simulink model "pre_lab"  (R2023b)
settings: Solver=ode4  StartTime=0.0  StopTime=5  FixedStep=1e-04  RelTol=1e-3
values from neighbouring files (symbols this model uses):
  CFP085 = (1/(2*pi*f))*(abs(Qc2)/(3*(Vc^2)))    [script.m]
  CFP095 = (1/(2*pi*f))*(abs(Qc3)/(3*(Vc^2)))    [script.m]
  CFP1 = (1/(2*pi*f))*(abs(Qc)/(3*(Vc^2)))    [script.m]
  f = 60    [script.m]
  L = XL/(omega)    (= 0.358098621957)    [script.m]
  r = 135    [script.m]
  Rc = 0.1    [script.m]
  Vl = 220    [script.m]
libraries: spsSeriesRLCBranchLib x18, spsThreePhaseBreakerLib x6, spsCurrentMeasurementLib x3, spsParallelRLCBranchLib x3, spsRMSLib x3, spsGroundLib x2, eePowerMeasurement x1, spsThreePhaseVIMeasurementLib x1, spsThreePhaseSourceLib x1, spsVoltageMeasurementLib x1, spspowerguiLib x1
settings Model: Creator=caugu  LastModifiedBy=caugu
settings ModelReferenceCC: EnableRefExpFcnMdlSchedulingChecks=on

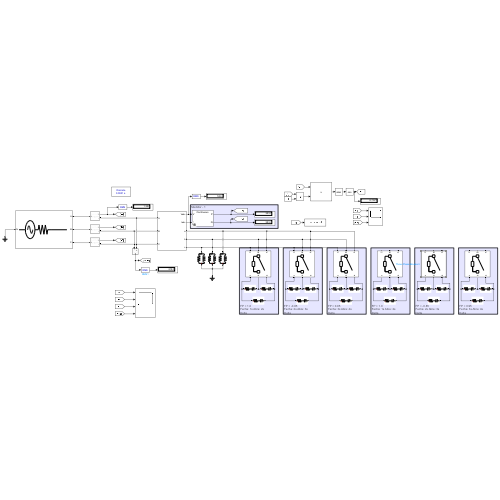
[thumbnail: Simulink's stored preview of the top-level diagram]
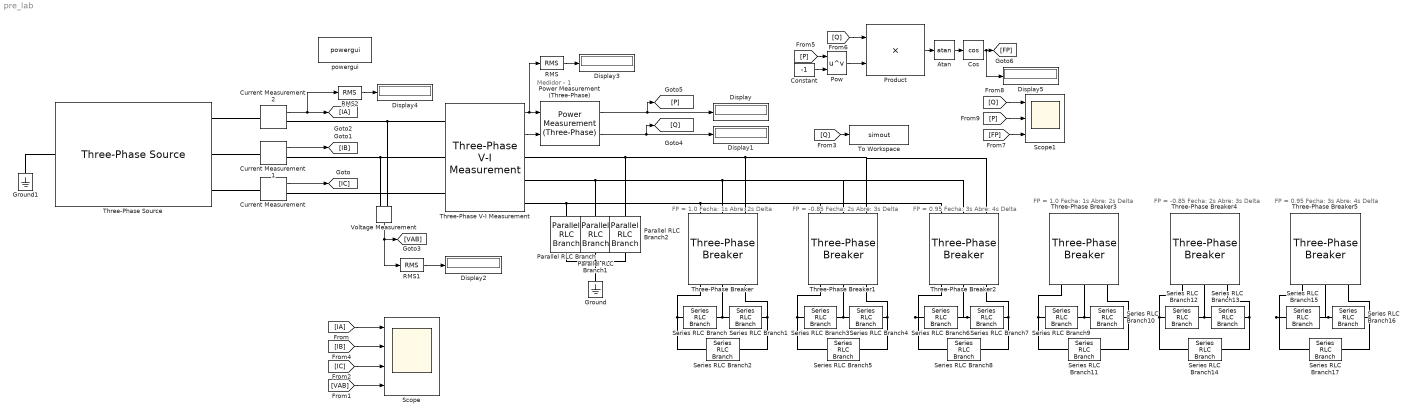
== system pre_lab ==
  note: FP = 1.0
      | Fecha: 1s Abre: 2s
      | Delta
  note: Medidor - 1
  note: FP = -0.85
      | Fecha: 2s Abre: 3s
      | Delta
  note: FP = 0.95
      | Fecha: 3s Abre: 4s
      | Delta
  note: FP = 1.0
      | Fecha: 1s Abre: 2s
      | Delta
  note: FP = -0.85
      | Fecha: 2s Abre: 3s
      | Delta
  note: FP = 0.95
      | Fecha: 3s Abre: 4s
      | Delta
  Atan : Trigonometry  Operator=atan
  Constant : Constant  Value=-1
  Cos : Trigonometry  Operator=cos
  Current Measurement : spsCurrentMeasurementLib/Current Measurement  PhasorSimulation=off  OutputType=Complex  PSBequivalent=0
  Current Measurement1 : spsCurrentMeasurementLib/Current Measurement  PhasorSimulation=off  OutputType=Complex  PSBequivalent=0
  Current Measurement2 : spsCurrentMeasurementLib/Current Measurement  PhasorSimulation=off  OutputType=Complex  PSBequivalent=0
  Display{,1..5} (6 alike) : Display
  Ground : spsGroundLib/Ground  LConnTagsString=a
  Ground1 : spsGroundLib/Ground  LConnTagsString=a
  Parallel RLC Branch : spsParallelRLCBranchLib/Parallel RLC Branch  LConnTagsString=a  RConnTagsString=__new0  BranchType=RL  Resistance=r  Inductance=L  SetiL0=off  InitialCurrent=0  Capacitance=1e-6  Setx0=off  InitialVoltage=0  Measurements=None
  Parallel RLC Branch1 : spsParallelRLCBranchLib/Parallel RLC Branch  LConnTagsString=a  RConnTagsString=__new0  BranchType=RL  Resistance=r  Inductance=L  SetiL0=off  InitialCurrent=0  Capacitance=1e-6  Setx0=off  InitialVoltage=0  Measurements=None
  Parallel RLC Branch2 : spsParallelRLCBranchLib/Parallel RLC Branch  LConnTagsString=a  RConnTagsString=__new0  BranchType=RL  Resistance=r  Inductance=L  SetiL0=off  InitialCurrent=0  Capacitance=1e-6  Setx0=off  InitialVoltage=0  Measurements=None
  Pow : Math  Operator=pow  SignedPower=on  RndMeth=Zero
  Power Measurement (Three-Phase) : eePowerMeasurement/Power Measurement (Three-Phase)  LabelModeActiveChoice=Continuous  F=60  K=[1]  Seq=Positive  Ts=0
  Product : Product
  RMS : spsRMSLib/RMS  TrueRMS=on  Freq=60  RMSInit=120  Ts=0
  RMS1 : spsRMSLib/RMS  TrueRMS=on  Freq=60  RMSInit=120  Ts=0
  RMS2 : spsRMSLib/RMS  TrueRMS=on  Freq=60  RMSInit=120  Ts=0
  Scope : Scope  NumInputPorts=4
  Scope1 : Scope  NumInputPorts=3
  Series RLC Branch{,1..2,9..11} (6 alike) : spsSeriesRLCBranchLib/Series RLC Branch  LConnTagsString=__new0  RConnTagsString=__new0  BranchType=RC  Resistance=Rc  Inductance=1e-3  SetiL0=off  InitialCurrent=0  Capacitance=CFP1  Setx0=off  InitialVoltage=0  Measurements=None
  Series RLC Branch{3..5,12..14} (6 alike) : spsSeriesRLCBranchLib/Series RLC Branch  LConnTagsString=__new0  RConnTagsString=__new0  BranchType=RC  Resistance=Rc  Inductance=1e-3  SetiL0=off  InitialCurrent=0  Capacitance=CFP085  Setx0=off  InitialVoltage=0  Measurements=None
  Series RLC Branch{6..8,15..17} (6 alike) : spsSeriesRLCBranchLib/Series RLC Branch  LConnTagsString=__new0  RConnTagsString=__new0  BranchType=RC  Resistance=Rc  Inductance=1e-3  SetiL0=off  InitialCurrent=0  Capacitance=CFP095  Setx0=off  InitialVoltage=0  Measurements=None
  Three-Phase V-I Measurement : spsThreePhaseVIMeasurementLib/Three-Phase V-I Measurement  VoltageMeasurement=phase-to-ground  SetLabelV=off  LabelV=Vabc  Vpu=off  VpuLL=off  CurrentMeasurement=yes  SetLabelI=off  LabelI=Iabc  Ipu=off  Pbase=100e6  Vbase=500e3  OutputType=Complex  PhasorSimulation=off  PSBequivalent=0
  Three-Phase Breaker : spsThreePhaseBreakerLib/Three-Phase Breaker  InitialState=open  SwitchA=on  SwitchB=on  SwitchC=on  SwitchTimes=[1 2]  External=off  BreakerResistance=0.01  SnubberResistance=1e6  SnubberCapacitance=inf  Measurements=None
  Three-Phase Breaker1 : spsThreePhaseBreakerLib/Three-Phase Breaker  InitialState=open  SwitchA=on  SwitchB=on  SwitchC=on  SwitchTimes=[2 3]  External=off  BreakerResistance=0.01  SnubberResistance=1e6  SnubberCapacitance=inf  Measurements=None
  Three-Phase Breaker2 : spsThreePhaseBreakerLib/Three-Phase Breaker  InitialState=open  SwitchA=on  SwitchB=on  SwitchC=on  SwitchTimes=[3 4]  External=off  BreakerResistance=0.01  SnubberResistance=1e6  SnubberCapacitance=inf  Measurements=None
  Three-Phase Breaker3 : spsThreePhaseBreakerLib/Three-Phase Breaker  InitialState=open  SwitchA=on  SwitchB=on  SwitchC=on  SwitchTimes=[1 2]  External=off  BreakerResistance=0.01  SnubberResistance=1e6  SnubberCapacitance=inf  Measurements=None
  Three-Phase Breaker4 : spsThreePhaseBreakerLib/Three-Phase Breaker  InitialState=open  SwitchA=on  SwitchB=on  SwitchC=on  SwitchTimes=[2 3]  External=off  BreakerResistance=0.01  SnubberResistance=1e6  SnubberCapacitance=inf  Measurements=None
  Three-Phase Breaker5 : spsThreePhaseBreakerLib/Three-Phase Breaker  InitialState=open  SwitchA=on  SwitchB=on  SwitchC=on  SwitchTimes=[3 4]  External=off  BreakerResistance=0.01  SnubberResistance=1e6  SnubberCapacitance=inf  Measurements=None
  Three-Phase Source : spsThreePhaseSourceLib/Three-Phase Source  InternalConnection=Yn  VoltagePhases=off  Voltage=Vl  PhaseAngle=0  Voltage_phases=[25e3 25e3 25e3]/sqrt(3)  PhaseAngles_phases=[0 -120 +120]  Frequency=f  NonIdealSource=on  SpecifyImpedance=off  Resistance=0.8929  Inductance=0  ShortCircuitLevel=100e6  BaseVoltage=25e3  XRratio=7  BusType=swing  Pref=10e3  Qref=0  Prefabc=[10e3, 10e3, 10e3]  Qrefabc=[0, 0, 0]  Qmin=-inf  Qmax=inf
  To Workspace : ToWorkspace  VariableName=simout  SaveFormat=Structure With Time  SampleTime=-1
  Voltage Measurement : spsVoltageMeasurementLib/Voltage Measurement  PhasorSimulation=off  OutputType=Complex  PSBequivalent=0
  powergui : spspowerguiLib/powergui  Priority=1  SimulationMode=Discrete  SampleTime=1e-4  frequency=60  Iterations=50  frequencyindice=0  Pbase=100e6  ErrMax=1e-4  UnitsV=kV  UnitsW=MW  buscounter=0  FunctionMessages=off  echomessages=off  EnableUseOfTLC=off  CurrentSourceSwitches=off  DisableSnubberDevices=off  DisableRonSwitches=off  DisableVfSwitches=off  DisplayEquations=off  AutomaticDiscreteSolvers=off  SolverType=Tustin/Backward Euler (TBE)  Interpol=off  ExternalGateDelay=off  methode=off  Ts=100  x0status=blocks  SPID=on  SwTol=0  HookPort=off  NonlinearTolerance=1e-4  nMaxIteration=100  ContinueOnMaxIteration=off  RestoreLinks=warning  ResistiveCurrentMeasurement=off  Frange=[0:2:500]  Ylog=off  Xlog=on  ShowGrid=off  save=off  variable=ZData  structure=0  ZoomFFT=off  StartTime=0.0  cycles=1  DisplayStyle=1  fundamental=60  FreqAxis=off  MaxFrequency=1000  frequencyindicesteady=1  RmsSteady=1  display=off
  wires:
  Current Measurement2/1 -> RMS2/1, [IA]
  Current Measurement1/1 -> [IB]
  Current Measurement/1 -> [IC]
  Voltage Measurement/1 -> RMS1/1, [VAB]
  Three-Phase V-I Measurement/1 -> RMS/1, Power Measurement (Three-Phase)/1
  Three-Phase V-I Measurement/2 -> Power Measurement (Three-Phase)/2
  Power Measurement (Three-Phase)/1 -> [P], Display/1
  Power Measurement (Three-Phase)/2 -> [Q], Display1/1
  [IA] -> Scope/1
  [VAB] -> Scope/4
  [IC] -> Scope/3
  [Q] -> To Workspace/1
  [IB] -> Scope/2
  RMS/1 -> Display3/1
  RMS1/1 -> Display2/1
  RMS2/1 -> Display4/1
  [FP] -> Scope1/3
  [Q] -> Scope1/1
  [P] -> Scope1/2
  Constant/1 -> Pow/2
  [P] -> Pow/1
  [Q] -> Product/1
  Pow/1 -> Product/2
  Product/1 -> Atan/1
  Atan/1 -> Cos/1
  Cos/1 -> Display5/1, [FP]
  connections:
  Current Measurement2/LConn1 -- Three-Phase Source/RConn1
  Three-Phase Source/RConn2 -- Current Measurement1/LConn1
  Three-Phase Source/RConn3 -- Current Measurement/LConn1
  Current Measurement2/RConn1 -- Voltage Measurement/LConn1 -- Three-Phase V-I Measurement/LConn1
  Current Measurement1/RConn1 -- Voltage Measurement/LConn2 -- Three-Phase V-I Measurement/LConn2
  Current Measurement/RConn1 -- Three-Phase V-I Measurement/LConn3
  Parallel RLC Branch2/RConn1 -- Three-Phase Breaker2/LConn1 -- Three-Phase Breaker1/LConn1 -- Three-Phase Breaker/LConn1 -- Three-Phase V-I Measurement/RConn1
  Three-Phase V-I Measurement/RConn2 -- Three-Phase Breaker2/LConn2 -- Three-Phase Breaker1/LConn2 -- Three-Phase Breaker/LConn2 -- Parallel RLC Branch1/RConn1
  Three-Phase V-I Measurement/RConn3 -- Three-Phase Breaker2/LConn3 -- Three-Phase Breaker1/LConn3 -- Three-Phase Breaker/LConn3 -- Parallel RLC Branch/RConn1
  Parallel RLC Branch1/LConn1 -- Parallel RLC Branch2/LConn1 -- Ground/LConn1 -- Parallel RLC Branch/LConn1
  Series RLC Branch1/LConn1 -- Three-Phase Breaker/RConn2 -- Series RLC Branch/RConn1
  Series RLC Branch2/RConn1 -- Series RLC Branch1/RConn1 -- Three-Phase Breaker/RConn1
  Series RLC Branch2/LConn1 -- Three-Phase Breaker/RConn3 -- Series RLC Branch/LConn1
  Three-Phase Source/LConn1 -- Ground1/LConn1
  Series RLC Branch4/LConn1 -- Series RLC Branch3/RConn1 -- Three-Phase Breaker1/RConn2
  Series RLC Branch5/RConn1 -- Three-Phase Breaker1/RConn1 -- Series RLC Branch4/RConn1
  Series RLC Branch5/LConn1 -- Series RLC Branch3/LConn1 -- Three-Phase Breaker1/RConn3
  Series RLC Branch6/RConn1 -- Series RLC Branch7/LConn1 -- Three-Phase Breaker2/RConn2
  Three-Phase Breaker2/RConn1 -- Series RLC Branch8/RConn1 -- Series RLC Branch7/RConn1
  Series RLC Branch6/LConn1 -- Series RLC Branch8/LConn1 -- Three-Phase Breaker2/RConn3
  Series RLC Branch10/LConn1 -- Series RLC Branch9/RConn1 -- Three-Phase Breaker3/RConn2
  Series RLC Branch11/RConn1 -- Three-Phase Breaker3/RConn1 -- Series RLC Branch10/RConn1
  Series RLC Branch11/LConn1 -- Series RLC Branch9/LConn1 -- Three-Phase Breaker3/RConn3
  Series RLC Branch13/LConn1 -- Three-Phase Breaker4/RConn2 -- Series RLC Branch12/RConn1
  Series RLC Branch14/RConn1 -- Series RLC Branch13/RConn1 -- Three-Phase Breaker4/RConn1
  Series RLC Branch14/LConn1 -- Three-Phase Breaker4/RConn3 -- Series RLC Branch12/LConn1
  Series RLC Branch15/RConn1 -- Three-Phase Breaker5/RConn2 -- Series RLC Branch16/LConn1
  Three-Phase Breaker5/RConn1 -- Series RLC Branch16/RConn1 -- Series RLC Branch17/RConn1
  Series RLC Branch15/LConn1 -- Three-Phase Breaker5/RConn3 -- Series RLC Branch17/LConn1
